simulink library "NeuroMuscularLibrary"  (R2014b)
settings: Solver=ode45  StartTime=0.0  StopTime=10.0  RelTol=1e-3
values from neighbouring files (symbols this model uses):
  c = 0.05    [BodyMechParams.m]
  c_jointstop = 0.3 / (pi/180)    (= 17.1887338539)    [BodyMechParams.m]
  DeltaThRef = 2e-3    (= 0.002)    [BodyMechParams.m]
  eref = 0.04    [BodyMechParams.m]
  footBallToAnkleDist = 0.16    [BodyMechParams.m]
  footBallToCenterDist = footLength/2    (= 0.1)    [BodyMechParams.m]
  footBallToHeelDist = footLength    (= 0.2)    [BodyMechParams.m]
  footCenterToCGDist = 0.14 - footBallToCenterDist    (= 0.04)    [BodyMechParams.m]
  footInertia = 0.005    [BodyMechParams.m]
  footLength = 0.2    [BodyMechParams.m]
  footMass = 1.25    [BodyMechParams.m]
  g = 9.80665    [BodyMechParams.m]
  groundTheta = [atan(diff(groundZ)./diff(groundX)), 0]    [generateGround.m]
  groundZ = groundZ * stepSize/(largestStep+eps)    [generateGround.m]
  hatHipToCenterDistLen = hatLength/2    (= 0.4)    [BodyMechParams.m]
  hatInertia = 3    [BodyMechParams.m]
  hatLeftHipToCenterDistWidth = .15    (= 0.15)    [BodyMechParams.m]
  hatLength = 0.8    [BodyMechParams.m]
  hatMass = 53.5    [BodyMechParams.m]
  hatThickness = 0.2    [BodyMechParams.m]
  hatWidth = 0.4    [BodyMechParams.m]
  K = 5    [BodyMechParams.m]
  k_gn = k_gz    (= 78453.2)    [BodyMechParams.m]
  k_gt = k_gz    (= 78453.2)    [BodyMechParams.m]
  k_pressure = hatMass * g / DeltaThRef    (= 262327.8875)    [BodyMechParams.m]
  loptGAS = 0.05    [BodyMechParams.m]
  loptGLU = 0.11    [BodyMechParams.m]
  loptHAM = 0.10    (= 0.1)    [BodyMechParams.m]
  loptHFL = 0.11    [BodyMechParams.m]
  loptSOL = 0.04    [BodyMechParams.m]
  loptTA = 0.06    [BodyMechParams.m]
  loptVAS = 0.08    [BodyMechParams.m]
  lslackGAS = 0.40    (= 0.4)    [BodyMechParams.m]
  lslackGLU = 0.13    [BodyMechParams.m]
  lslackHAM = 0.31    [BodyMechParams.m]
  lslackHFL = 0.10    (= 0.1)    [BodyMechParams.m]
  lslackSOL = 0.26    [BodyMechParams.m]
  lslackTA = 0.24    [BodyMechParams.m]
  lslackVAS = 0.23    [BodyMechParams.m]
  mu_slide = 0.8    [BodyMechParams.m]
  mu_stick = 0.9    [BodyMechParams.m]
  N = 1.5    [BodyMechParams.m]    (also in cmaes.m = size(x,1))
  phimaxGASa = 20*pi/180    (= 0.349065850399)    [BodyMechParams.m]
  phimaxGASk = 40*pi/180    (= 0.698131700798)    [BodyMechParams.m]
  phimaxHAMk = 0*pi/180    (= 0)    [BodyMechParams.m]
  phimaxSOL = 20*pi/180    (= 0.349065850399)    [BodyMechParams.m]
  phimaxTA = -10*pi/180    (= -0.174532925199)    [BodyMechParams.m]
  phimaxVAS = 15*pi/180    (= 0.261799387799)    [BodyMechParams.m]
  phirefGASa = -10*pi/180    (= -0.174532925199)    [BodyMechParams.m]
  phirefGASk = 15*pi/180    (= 0.261799387799)    [BodyMechParams.m]
  phirefGLU = -30*pi/180    (= -0.523598775598)    [BodyMechParams.m]
  phirefHAMh = -25*pi/180    (= -0.436332312999)    [BodyMechParams.m]
  phirefHAMk = 0*pi/180    (= 0)    [BodyMechParams.m]
  phirefHFL = 0*pi/180    (= 0)    [BodyMechParams.m]
  phirefSOL = -10*pi/180    (= -0.174532925199)    [BodyMechParams.m]
  phirefTA = 20*pi/180    (= 0.349065850399)    [BodyMechParams.m]
  phirefVAS = 55*pi/180    (= 0.959931088597)    [BodyMechParams.m]
  rGASa = 0.05    [BodyMechParams.m]
  rGASk = 0.05    [BodyMechParams.m]
  rGLU = 0.10    (= 0.1)    [BodyMechParams.m]
  rHAMh = 0.08    [BodyMechParams.m]
  rHAMk = 0.05    [BodyMechParams.m]
  rHFL = 0.10    (= 0.1)    [BodyMechParams.m]
  rhoGASa = 0.7    [BodyMechParams.m]
  rhoGASk = 0.7    [BodyMechParams.m]
  rhoGLU = 0.5    [BodyMechParams.m]
  rhoHAMh = 0.7    [BodyMechParams.m]
  rhoHAMk = 0.7    [BodyMechParams.m]
  rhoHFL = 0.5    [BodyMechParams.m]
  rhoSOL = 0.5    [BodyMechParams.m]
  rhoTA = 0.7    [BodyMechParams.m]
  rhoVAS = 0.7    [BodyMechParams.m]
  rSOL = 0.05    [BodyMechParams.m]
  rTA = 0.04    [BodyMechParams.m]
  rVAS = 0.06    [BodyMechParams.m]
  s = x(1:N-1,:).^2 + x(2:N,:).^2    [cmaes.m]
  shankAnkleToCenterDist = shankLength/2    (= 0.25)    [BodyMechParams.m]
  shankAnkleToKneeDist = shankLength    (= 0.5)    [BodyMechParams.m]
  shankCenterToCGDist = 0.3 - shankAnkleToCenterDist    (= 0.05)    [BodyMechParams.m]
  shankInertia = 0.05    [BodyMechParams.m]
  shankLength = 0.5    [BodyMechParams.m]
  shankMass = 3.5    [BodyMechParams.m]
  tau = 0.01    [BodyMechParams.m]
  thighCenterToCGDist = 0.3 - thighKneeToCenterDist    (= 0.05)    [BodyMechParams.m]
  thighInertia = 0.15    [BodyMechParams.m]
  thighKneeToCenterDist = thighLength/2    (= 0.25)    [BodyMechParams.m]
  thighKneeToHipDist = thighLength    (= 0.5)    [BodyMechParams.m]
  thighLength = 0.5    [BodyMechParams.m]
  thighMass = 8.5    [BodyMechParams.m]
  v_gn_max = v_gz_max    (= 0.03)    [BodyMechParams.m]
  v_gt_max = v_gz_max    (= 0.03)    [BodyMechParams.m]
  v_max_pressure = 0.5    [BodyMechParams.m]
  vLimit = 0.01    [BodyMechParams.m]
  w = 0.56    [BodyMechParams.m]    (also in cmaes.m = ones(size(x,1)))
  w_max_jointstop = 1 * pi/180    (= 0.0174532925199)    [BodyMechParams.m]
undefined symbols (not defined in the file or in its folder): ankleBackDriveGain, ankleDgain, ankleFilterPID, ankleFilterSEA, ankleGearEff, ankleGearRatio, ankleIgain, ankleInitialAngle, ankleInputMass, ankleParallelSpringDamping, ankleParallelSpringOffset, ankleParallelSpringStiffness, anklePgain, ankleSEADamping, ankleSEAStiffness, ankleTendonMass, deltaLegAngleThr, footMassp, FourBarL1, FourBarL3, GainGAS, GainGLU, GainHAM, GainKneeOverExt, GainSOL, GainSOLTA, GainTA, GainVAS, hipDGain, hipPGain, Kglu, kneeAngleOffset, kneeBackDriveGain, kneeDgain, kneeExtendGain, kneeFilterPID, kneeFilterSEA, kneeFlexGain, kneeGearEff, kneeGearRatio, kneeHoldGain1, kneeHoldGain2, kneeIgain, kneeInitialAngle, kneePgain, kneeSEADamping, kneeSEAStiffness, kneeStatorMass, kneeStopGain, legAngleFilter, legAngleSpeedMax, legLengthClr, motorBackEMF, motorInductance, motorMaxCurrent, motorMaxVoltage, motorResistance, motorRotorInertia, motorRotorMass, motorTorsionalConst ... (+19)
undefined symbols (not defined in the file): ankleCJointstop, ankleIntCoulomb, ankleIntDamping, ankleIntStatic, anklePlantarLimit, ankleWMaxJointstop, dryFrictionDamping, dryFrictionStiffness, dryFrictionVelThresh, FmaxGLU, FT_GLU, kneeCJointstop, kneeExtCoulomb, kneeExtDamping, kneeExtStatic, kneeIntCoulomb, kneeIntDamping, kneeIntStatic, kneeWMaxJointstop, phiKneeUpLimit, RGainGAS, RGainGLU, RGainHAM, RGainHAMCut, RGainKneeOverExt, RGainSOL, RGainSOLTA, RGainTA, RGainVAS, RhipDGain, RhipPGain, RKglu, RkneeExtendGain, RkneeFlexGain, RkneeHoldGain1, RkneeHoldGain2, RkneeStopGain, RlegAngleFilter, RlegLengthClr, RPosGainGG, RSpeedGainGG
libraries: sm_lib x90, nesl_utility x44, simulink x18, dspswit3 x10, NeuroMuscularLibrary x8, simulink_extras x2
(part 4 of 5)

== system NeuroMuscularLibrary/Full Prosthesis/Ankle SEA Control ==
  Motor Speed : Inport
  Load Acceleration : Inport  Port=2
  Measured Torque : Inport  Port=3
  Desired Ankle Torque : Inport  Port=4
  Parallel Spring Torque : Inport  Port=5
  Ankle Input Angle : Inport  Port=6
  Tendon Angle : Inport  Port=7
  Ankle Angle : Inport  Port=8
  4 bar ratio : Subsystem
  Divide : Product  Inputs=*/
  Feed Forward : Subsystem
  PID Controller : simulink/Continuous/PID Controller  Controller=PD  TimeDomain=Continuous-time  SampleTime=-1  IntegratorMethod=Forward Euler  FilterMethod=Forward Euler  Form=Parallel  P=anklePgain  I=ankleIgain  D=ankleDgain  N=ankleFilterPID  InitialConditionSource=internal  InitialConditionForIntegrator=0  InitialConditionForFilter=0  ExternalReset=none  LimitOutput=off  UpperSaturationLimit=inf  LowerSaturationLimit=-inf  LinearizeAsGain=on  AntiWindupMode=none  Kb=1  TrackingMode=off  Kt=1  PParamMin=[]  PParamMax=[]  IParamMin=[]  IParamMax=[]  DParamMin=[]  DParamMax=[]  NParamMin=[]  NParamMax=[]  KbParamMin=[]  KbParamMax=[]  KtParamMin=[]  KtParamMax=[]  POutMin=[]  POutMax=[]  IOutMin=[]  IOutMax=[]  DOutMin=[]  DOutMax=[]  NOutMin=[]  NOutMax=[]  KbOutMin=[]  KbOutMax=[]  KtOutMin=[]  KtOutMax=[]  IntegratorOutMin=[]  IntegratorOutMax=[]  FilterOutMin=[]  FilterOutMax=[]  SumOutMin=[]  SumOutMax=[]  SumI1OutMin=[]  SumI1OutMax=[]  SumI2OutMin=[]  SumI2OutMax=[]  SumI3OutMin=[]  SumI3OutMax=[]  SumDOutMin=[]  SumDOutMax=[]  SaturationOutMin=[]  SaturationOutMax=[]  IntegratorContinuousStateAttributes=''  IntegratorStateMustResolveToSignalObject=off  IntegratorRTWStateStorageClass=Auto  FilterContinuousStateAttributes=''  FilterStateMustResolveToSignalObject=off  FilterRTWStateStorageClass=Auto  DifferentiatorICPrevScaledInput=0  DifferentiatorOutMin=[]  DifferentiatorOutMax=[]  UseFilter=on
  Saturation1 : Saturate  UpperLimit=motorMaxVoltage  LowerLimit=-motorMaxVoltage  ZeroCross=off
  Sum : Sum  Inputs=|+-
  Sum1 : Sum  Inputs=+-|
  Sum2 : Sum  Inputs=|+-
  Motor Voltage : Outport
  Desired Actuator Torque : Outport  Port=2
  wires:
  Divide/1 -> Sum/1, Feed Forward/3(Desired Actuator Torque), Desired Actuator Torque/1  "Desired Actuator"
  Sum2/1 -> Divide/1
  Saturation1/1 -> Motor Voltage/1
  Sum1/1 -> Saturation1/1
  Load Acceleration/1 -> Feed Forward/2(Load Acceleration)
  Ankle Input Angle/1 -> 4 bar ratio/1(Ankle Input Angle)
  Tendon Angle/1 -> 4 bar ratio/2(Tendon Angle)
  Ankle Angle/1 -> 4 bar ratio/3(Ankle Angle)
  Measured Torque/1 -> Sum/2
  Sum/1 -> PID Controller/1
  4 bar ratio/1(ratio) -> Divide/2
  Motor Speed/1 -> Feed Forward/1(Motor Speed)
  Feed Forward/1(Computed Motor Voltage) -> Sum1/1
  Desired Ankle Torque/1 -> Sum2/1
  Parallel Spring Torque/1 -> Sum2/2
  PID Controller/1 -> Sum1/2

== system NeuroMuscularLibrary/Full Prosthesis/Ankle Tendon ==
  CG : sm_lib/Frames and Transforms/Reference Frame  BlockFunction=simmechanics.library.frames_transforms.reference_frame
  PS-Simulink Converter : nesl_utility/PS-Simulink Converter  PhysicalDomain=network_engine_domain  SubClassName=ps_output  LeftPortType=input  RightPortType=output  PseudoPeriodic=off  Frequencies=[]  Unit=1  AffineConversion=off
  Revolute Joint : sm_lib/Joints/Revolute Joint  SenseConstraintForce=off  SenseConstraintForceX=off  SenseConstraintForceY=off  SenseConstraintForceZ=off  SenseConstraintTorque=off  SenseConstraintTorqueX=off  SenseConstraintTorqueY=off  SenseConstraintTorqueZ=off  SenseTotalForce=off  SenseTotalForceX=off  SenseTotalForceY=off  SenseTotalForceZ=off  SenseTotalTorque=off  SenseTotalTorqueX=off  SenseTotalTorqueY=off  SenseTotalTorqueZ=off  CompositeWrenchDir=FollowerOnBase  CompositeWrenchFrame=BaseFrame  EquilibriumPosition=0  EquilibriumPositionUnits=deg  SpringStiffness=0  SpringStiffnessUnits=N*m/deg  DampingCoefficient=0  DampingCoefficientUnits=N*m/(deg/s)  TorqueActuationMode=NoTorque  MotionActuationMode=ComputedMotion  SensePosition=on  SenseVelocity=off  SenseAcceleration=off  SenseTorqueForce=off  PositionTargetValue=0  PositionTargetValueUnits=deg  PositionTargetSpecify=off  PositionTargetPriority=High  VelocityTargetValue=0  VelocityTargetValueUnits=deg/s  VelocityTargetSpecify=off  VelocityTargetPriority=High  BlockFunction=simmechanics.library.joints.revolute_joint
  Revolute Joint1 : sm_lib/Joints/Revolute Joint  SenseConstraintForce=off  SenseConstraintForceX=off  SenseConstraintForceY=off  SenseConstraintForceZ=off  SenseConstraintTorque=off  SenseConstraintTorqueX=off  SenseConstraintTorqueY=off  SenseConstraintTorqueZ=off  SenseTotalForce=off  SenseTotalForceX=off  SenseTotalForceY=off  SenseTotalForceZ=off  SenseTotalTorque=off  SenseTotalTorqueX=off  SenseTotalTorqueY=off  SenseTotalTorqueZ=off  CompositeWrenchDir=FollowerOnBase  CompositeWrenchFrame=BaseFrame  EquilibriumPosition=0  EquilibriumPositionUnits=deg  SpringStiffness=0  SpringStiffnessUnits=N*m/deg  DampingCoefficient=0  DampingCoefficientUnits=N*m/(deg/s)  TorqueActuationMode=NoTorque  MotionActuationMode=ComputedMotion  SensePosition=off  SenseVelocity=off  SenseAcceleration=off  SenseTorqueForce=off  PositionTargetValue=0  PositionTargetValueUnits=deg  PositionTargetSpecify=off  PositionTargetPriority=High  VelocityTargetValue=0  VelocityTargetValueUnits=deg/s  VelocityTargetSpecify=off  VelocityTargetPriority=High  BlockFunction=simmechanics.library.joints.revolute_joint
  Shank : sm_lib/Body Elements/Solid  InertiaType=Custom  Mass=ankleTendonMass  MassUnits=g  CenterOfMass=ankleTendonCG  CenterOfMassUnits=mm  MomentsOfInertia=ankleTendonMomentOfInertia  MomentsOfInertiaUnits=g*cm^2  ProductsOfInertia=ankleTendonProductOfInertia  ProductsOfInertiaUnits=g*cm^2  DensityBased=on  Density=1000  DensityUnits=kg/(m^3)  GraphicType=FromGeometry  MarkerShape=Sphere  MarkerSize=10  MarkerSizeUnits=m  GraphicVisPropType=SimpleVisualProperties  GraphicDiffuseColor=[0.5 0.5 0.5]  GraphicSpecularColor=[0.5 0.5 0.5 1.0]  GraphicAmbientColor=[0.15 0.15 0.15 1.0]  GraphicEmissiveColor=[0.0 0.0 0.0 1.0]  GraphicShininess=75  GraphicOpacity=1.0  GeometryShape=FromFile  RectangleSize=[1 1]  RectangleSizeUnits=m  BrickDimensions=[1 1 1]  BrickDimensionUnits=m  CylinderRadius=1  CylinderRadiusUnits=m  CylinderLength=1  CylinderLengthUnits=m  SphereRadius=1  SphereRadiusUnits=m  EllipsoidRadii=[1 1 1]  EllipsoidRadiiUnits=m  ExtrusionCrossSection=[1 1; -1 1; -1 -1; 1 -1]  ExtrusionCrossSectionUnits=m  ExtrusionLength=1  ExtrusionLengthUnits=m  PolygonNumSides=3  PolygonOuterRadius=1  PolygonOuterRadiusUnits=m  ExtGeomFileType=STL  ExtGeomFileName=ankleTendon.STL  ExtGeomFileUnits=mm  RevolutionCrossSection=[1 1; 1 -1; 2 -1; 2 1]  RevolutionCrossSectionUnits=m  RevolutionExtent=Full  RevolutionAngle=180  RevolutionAngleUnits=deg  BlockFunction=simmechanics.library.body_elements.solid
  To CG : sm_lib/Frames and Transforms/Rigid Transform  TranslationMethod=Cartesian  TranslationLengthUnit=mm  TranslationStandardAxis=-Z  TranslationStandardOffset=1.5  TranslationCartesianOffset=ankleTendonCG  TranslationROffset=0  TranslationROffsetUnits=m  TranslationZOffset=0  TranslationZOffsetUnits=m  TranslationThetaOffset=0  TranslationThetaOffsetUnits=deg  RotationMethod=None  RotationAngleUnits=deg  RotationStandardAxis=+Z  RotationAngle=0  RotationArbitraryAxis=[0 0 1]  FollAlignAxisA=+X  BaseAlignAxisA=+Y  FollAlignAxisB=+Y  BaseAlignAxisB=+Z  RotationMatrix=[1 0 0; 0 1 0; 0 0 1]  BlockFunction=simmechanics.library.frames_transforms.rigid_transform
  To Foot : sm_lib/Frames and Transforms/Rigid Transform  TranslationMethod=Cartesian  TranslationLengthUnit=mm  TranslationStandardAxis=-Y  TranslationStandardOffset=445.61  TranslationCartesianOffset=[0, -328.8, 0]  TranslationROffset=0  TranslationROffsetUnits=m  TranslationZOffset=0  TranslationZOffsetUnits=m  TranslationThetaOffset=0  TranslationThetaOffsetUnits=deg  RotationMethod=None  RotationAngleUnits=deg  RotationStandardAxis=+Z  RotationAngle=0  RotationArbitraryAxis=[0 0 1]  FollAlignAxisA=+X  BaseAlignAxisA=+Y  FollAlignAxisB=+Y  BaseAlignAxisB=+Z  RotationMatrix=[1 0 0; 0 1 0; 0 0 1]  BlockFunction=simmechanics.library.frames_transforms.rigid_transform
  " Ankle Input Joint" : PMIOPort  Port=1  Side=Left
  Foot : PMIOPort  Port=2  Side=Right
  Angle : Outport
  wires:
  PS-Simulink Converter/1 -> Angle/1
  connections:
  CG/RConn1 -- To CG/RConn1
  To Foot/LConn1 -- Revolute Joint/RConn1 -- To CG/LConn1 -- Shank/RConn1
  Revolute Joint/LConn1 -- " Ankle Input Joint"/RConn1
  Revolute Joint1/LConn1 -- To Foot/RConn1
  Foot/RConn1 -- Revolute Joint1/RConn1
  Revolute Joint/RConn2 -- PS-Simulink Converter/LConn1

== system NeuroMuscularLibrary/Full Prosthesis/Foot ==
  CG : sm_lib/Frames and Transforms/Reference Frame  BlockFunction=simmechanics.library.frames_transforms.reference_frame
  Shank : sm_lib/Body Elements/Solid  InertiaType=Custom  Mass=footMassp  MassUnits=g  CenterOfMass=footCG  CenterOfMassUnits=mm  MomentsOfInertia=footMomentOfInertia  MomentsOfInertiaUnits=g*cm^2  ProductsOfInertia=footProductOfInertia  ProductsOfInertiaUnits=g*cm^2  DensityBased=on  Density=1000  DensityUnits=kg/(m^3)  GraphicType=FromGeometry  MarkerShape=Sphere  MarkerSize=10  MarkerSizeUnits=m  GraphicVisPropType=SimpleVisualProperties  GraphicDiffuseColor=[0.5 0.5 0.5]  GraphicSpecularColor=[0.5 0.5 0.5 1.0]  GraphicAmbientColor=[0.15 0.15 0.15 1.0]  GraphicEmissiveColor=[0.0 0.0 0.0 1.0]  GraphicShininess=75  GraphicOpacity=1.0  GeometryShape=FromFile  RectangleSize=[1 1]  RectangleSizeUnits=m  BrickDimensions=[1 1 1]  BrickDimensionUnits=m  CylinderRadius=1  CylinderRadiusUnits=m  CylinderLength=1  CylinderLengthUnits=m  SphereRadius=1  SphereRadiusUnits=m  EllipsoidRadii=[1 1 1]  EllipsoidRadiiUnits=m  ExtrusionCrossSection=[1 1; -1 1; -1 -1; 1 -1]  ExtrusionCrossSectionUnits=m  ExtrusionLength=1  ExtrusionLengthUnits=m  PolygonNumSides=3  PolygonOuterRadius=1  PolygonOuterRadiusUnits=m  ExtGeomFileType=STL  ExtGeomFileName=foot.STL  ExtGeomFileUnits=mm  RevolutionCrossSection=[1 1; 1 -1; 2 -1; 2 1]  RevolutionCrossSectionUnits=m  RevolutionExtent=Full  RevolutionAngle=180  RevolutionAngleUnits=deg  BlockFunction=simmechanics.library.body_elements.solid
  To Ball : sm_lib/Frames and Transforms/Rigid Transform  TranslationMethod=Cartesian  TranslationLengthUnit=mm  TranslationStandardAxis=-Y  TranslationStandardOffset=445.61  TranslationCartesianOffset=[165, -63, 0]  TranslationROffset=0  TranslationROffsetUnits=m  TranslationZOffset=0  TranslationZOffsetUnits=m  TranslationThetaOffset=0  TranslationThetaOffsetUnits=deg  RotationMethod=None  RotationAngleUnits=deg  RotationStandardAxis=+Z  RotationAngle=0  RotationArbitraryAxis=[0 0 1]  FollAlignAxisA=+X  BaseAlignAxisA=+Y  FollAlignAxisB=+Y  BaseAlignAxisB=+Z  RotationMatrix=[1 0 0; 0 1 0; 0 0 1]  BlockFunction=simmechanics.library.frames_transforms.rigid_transform
  To CG : sm_lib/Frames and Transforms/Rigid Transform  TranslationMethod=Cartesian  TranslationLengthUnit=mm  TranslationStandardAxis=-Z  TranslationStandardOffset=1.5  TranslationCartesianOffset=footCG  TranslationROffset=0  TranslationROffsetUnits=m  TranslationZOffset=0  TranslationZOffsetUnits=m  TranslationThetaOffset=0  TranslationThetaOffsetUnits=deg  RotationMethod=None  RotationAngleUnits=deg  RotationStandardAxis=+Z  RotationAngle=0  RotationArbitraryAxis=[0 0 1]  FollAlignAxisA=+X  BaseAlignAxisA=+Y  FollAlignAxisB=+Y  BaseAlignAxisB=+Z  RotationMatrix=[1 0 0; 0 1 0; 0 0 1]  BlockFunction=simmechanics.library.frames_transforms.rigid_transform
  To Heel : sm_lib/Frames and Transforms/Rigid Transform  TranslationMethod=Cartesian  TranslationLengthUnit=mm  TranslationStandardAxis=-Y  TranslationStandardOffset=445.61  TranslationCartesianOffset=[-60, -63, 0]  TranslationROffset=0  TranslationROffsetUnits=m  TranslationZOffset=0  TranslationZOffsetUnits=m  TranslationThetaOffset=0  TranslationThetaOffsetUnits=deg  RotationMethod=None  RotationAngleUnits=deg  RotationStandardAxis=+Z  RotationAngle=0  RotationArbitraryAxis=[0 0 1]  FollAlignAxisA=+X  BaseAlignAxisA=+Y  FollAlignAxisB=+Y  BaseAlignAxisB=+Z  RotationMatrix=[1 0 0; 0 1 0; 0 0 1]  BlockFunction=simmechanics.library.frames_transforms.rigid_transform
  To Tendon : sm_lib/Frames and Transforms/Rigid Transform  TranslationMethod=Cartesian  TranslationLengthUnit=mm  TranslationStandardAxis=-Y  TranslationStandardOffset=445.61  TranslationCartesianOffset=[-81, -16.3, 0]  TranslationROffset=0  TranslationROffsetUnits=m  TranslationZOffset=0  TranslationZOffsetUnits=m  TranslationThetaOffset=0  TranslationThetaOffsetUnits=deg  RotationMethod=None  RotationAngleUnits=deg  RotationStandardAxis=+Z  RotationAngle=0  RotationArbitraryAxis=[0 0 1]  FollAlignAxisA=+X  BaseAlignAxisA=+Y  FollAlignAxisB=+Y  BaseAlignAxisB=+Z  RotationMatrix=[1 0 0; 0 1 0; 0 0 1]  BlockFunction=simmechanics.library.frames_transforms.rigid_transform
  " Ankle Input Joint" : PMIOPort  Port=1  Side=Right
  Tendon Bearing : PMIOPort  Port=2  Side=Left
  Ball : PMIOPort  Port=3  Side=Left
  Heel : PMIOPort  Port=4  Side=Right
  connections:
  Tendon Bearing/RConn1 -- To Tendon/RConn1
  CG/RConn1 -- To CG/RConn1
  To Tendon/LConn1 -- " Ankle Input Joint"/RConn1 -- Shank/RConn1 -- To CG/LConn1 -- To Heel/LConn1 -- To Ball/LConn1
  Ball/RConn1 -- To Ball/RConn1
  Heel/RConn1 -- To Heel/RConn1

== system NeuroMuscularLibrary/Full Prosthesis/Harmonic Drive// Series Elastic Actuator ==
  Motor Speed : Inport
  Motor Angle : Inport  Port=2
  Motor Torque : Inport  Port=3
  Load Angle : Inport  Port=4
  Load Speed : Inport  Port=5
  Add : Sum
  Damping : Gain  Gain=kneeSEADamping
  Gain : Gain  Gain=-1
  Mux : Mux  Inputs=2
  Ratio1 : Gain  Gain=1/kneeGearRatio
  Ratio2 : Gain  Gain=1/kneeGearRatio
  Ratio3 : Gain  Gain=1/kneeGearRatio
  Ratio4 : Gain  Gain=1/kneeGearEff
  Scope : Scope
  Stiffness : Gain  Gain=kneeSEAStiffness
  Sum : Sum  Inputs=|++
  Sum1 : Sum  Inputs=|++
  Sum2 : Sum  Inputs=++|
  Torque on Motor : Outport
  " Torque on Load" : Outport  Port=2
  wires:
  Mux/1 -> Scope/1
  Load Speed/1 -> Sum2/2
  Ratio3/1 -> Sum2/1
  Motor Torque/1 -> Sum1/2
  Ratio2/1 -> Ratio4/1
  Load Angle/1 -> Sum/1
  Add/1 -> Gain/1  "External Torque"
  Ratio1/1 -> Sum/2
  Sum1/1 -> Torque on Motor/1
  Stiffness/1 -> Add/2, Mux/1
  Sum/1 -> Stiffness/1
  Damping/1 -> Add/1, Mux/2
  Sum2/1 -> Damping/1
  Motor Speed/1 -> Ratio3/1
  Motor Angle/1 -> Ratio1/1
  Ratio4/1 -> Sum1/1
  Gain/1 -> " Torque on Load"/1, Ratio2/1

== system NeuroMuscularLibrary/Full Prosthesis/Harmonic Drive// Series Elastic Actuator1 ==
  Motor Speed : Inport
  Motor Angle : Inport  Port=2
  Motor Torque : Inport  Port=3
  Load Angle : Inport  Port=4
  Load Speed : Inport  Port=5
  Add : Sum
  Damping : Gain  Gain=ankleSEADamping
  Gain : Gain  Gain=-1
  Ratio1 : Gain  Gain=1/ankleGearRatio
  Ratio2 : Gain  Gain=1/ankleGearRatio
  Ratio3 : Gain  Gain=1/ankleGearRatio
  Ratio4 : Gain  Gain=1/ankleGearEff
  Stiffness : Gain  Gain=ankleSEAStiffness
  Sum : Sum  Inputs=|++
  Sum1 : Sum  Inputs=|++
  Sum2 : Sum  Inputs=++|
  Torque on Motor : Outport
  Torque on Load : Outport  Port=2
  wires:
  Gain/1 -> Torque on Load/1, Ratio2/1
  Load Speed/1 -> Sum2/2
  Ratio3/1 -> Sum2/1
  Motor Torque/1 -> Sum1/2
  Ratio2/1 -> Ratio4/1
  Load Angle/1 -> Sum/1
  Add/1 -> Gain/1  "External Torque"
  Ratio1/1 -> Sum/2
  Sum1/1 -> Torque on Motor/1
  Stiffness/1 -> Add/2
  Sum/1 -> Stiffness/1
  Damping/1 -> Add/1
  Sum2/1 -> Damping/1
  Motor Speed/1 -> Ratio3/1
  Motor Angle/1 -> Ratio1/1
  Ratio4/1 -> Sum1/1

== system NeuroMuscularLibrary/Full Prosthesis/Knee Joint ==
  External Torque : Inport
  Add : Sum  Inputs=+++
  Friction : Subsystem  Commented=on  mask{Fs=kneeExtStatic, Fc=kneeExtCoulomb, sigma0=dryFrictionStiffness, sigma1=dryFrictionDamping, v_s=dryFrictionVelThresh, Fv=kneeExtDamping}
      mask prompts: Fs "Static Friction"; Fc "Colulomb Friction"; sigma0 "Dry Friction Stiffness"; sigma1 "Dry Friction Damping"; v_s "Velocity Threshold"; Fv "Viscous Friction"
  Knee Joint : sm_lib/Joints/Revolute Joint  SenseConstraintForce=off  SenseConstraintForceX=off  SenseConstraintForceY=off  SenseConstraintForceZ=off  SenseConstraintTorque=off  SenseConstraintTorqueX=off  SenseConstraintTorqueY=off  SenseConstraintTorqueZ=off  SenseTotalForce=off  SenseTotalForceX=off  SenseTotalForceY=off  SenseTotalForceZ=off  SenseTotalTorque=off  SenseTotalTorqueX=off  SenseTotalTorqueY=off  SenseTotalTorqueZ=off  CompositeWrenchDir=FollowerOnBase  CompositeWrenchFrame=BaseFrame  EquilibriumPosition=0  EquilibriumPositionUnits=deg  SpringStiffness=0  SpringStiffnessUnits=N*m/rad  DampingCoefficient=0  DampingCoefficientUnits=N*m/(rad/s)  TorqueActuationMode=InputTorque  MotionActuationMode=ComputedMotion  SensePosition=on  SenseVelocity=on  SenseAcceleration=on  SenseTorqueForce=off  PositionTargetValue=kneeInitialAngle  PositionTargetValueUnits=rad  PositionTargetSpecify=on  PositionTargetPriority=High  VelocityTargetValue=0  VelocityTargetValueUnits=deg/s  VelocityTargetSpecify=off  VelocityTargetPriority=High  BlockFunction=simmechanics.library.joints.revolute_joint
  Knee Plantarflexion Limit : Subsystem  mask{phiUpLimit=0, ext=1, c_jointstop=kneeCJointstop, w_max_jointstop=kneeWMaxJointstop}
      mask prompts: phiUpLimit "Upper Limit [rad]"; ext "Extension values are positive or negative?"; c_jointstop "Stiffness"; w_max_jointstop "Max retraction speed"
      mask help:
      | This block implements a hard joint limit that will prevent the joint from extending past the specified upper limit.
      |
      | Used for the knee and hip joints.
  PS-Simulink Converter1 : nesl_utility/PS-Simulink Converter  PhysicalDomain=network_engine_domain  SubClassName=ps_output  LeftPortType=input  RightPortType=output  PseudoPeriodic=off  Frequencies=[]  Unit=rad/s^2  AffineConversion=off
  PS-Simulink Converter2 : nesl_utility/PS-Simulink Converter  PhysicalDomain=network_engine_domain  SubClassName=ps_output  LeftPortType=input  RightPortType=output  PseudoPeriodic=off  Frequencies=[]  Unit=rad  AffineConversion=off
  PS-Simulink Converter3 : nesl_utility/PS-Simulink Converter  PhysicalDomain=network_engine_domain  SubClassName=ps_output  LeftPortType=input  RightPortType=output  PseudoPeriodic=off  Frequencies=[]  Unit=rad/s  AffineConversion=off
  Scope : Scope  NumInputPorts=2
      settings: TimeRange=5  YMin=-0.5~-4  YMax=0.5~5  SaveName=ScopeData4
  Simulink-PS Converter : nesl_utility/Simulink-PS Converter  PhysicalDomain=network_engine_domain  SubClassName=ps_input  LeftPortType=input  RightPortType=output  PseudoPeriodic=off  Frequencies=[]  NoiseDistribution=none  NoiseParameters=[]  Unit=N*m  AffineConversion=off  InputFiltering=off  SimscapeFilterOrder=1  InputFilterTimeConstant=0.001  UdotUserProvided=1
  Knee Stator : PMIOPort  Port=1  Side=Right
  Shank : PMIOPort  Port=2  Side=Left
  Shank Angle : Outport
  Shank Speed : Outport  Port=2
  Shank Acceleration : Outport  Port=3
  Actual Torque : Outport  Port=4
  Knee Stop Torque : Outport  Port=5
  wires:
  Knee Plantarflexion Limit/1(M_stop [Nm]) -> Add/3, Knee Stop Torque/1
  PS-Simulink Converter2/1 -> Knee Plantarflexion Limit/1(phi [rad]), Shank Angle/1
  PS-Simulink Converter3/1 -> Knee Plantarflexion Limit/2(dphi [rad/s]), Scope/2, Friction/1(Velocity), Shank Speed/1
  PS-Simulink Converter1/1 -> Shank Acceleration/1
  Add/1 -> Actual Torque/1, Simulink-PS Converter/1
  External Torque/1 -> Add/1
  Friction/1(Friction Force) -> Add/2, Scope/1
  connections:
  Knee Joint/LConn1 -- Knee Stator/RConn1
  Knee Joint/RConn1 -- Shank/RConn1
  Knee Joint/RConn3 -- PS-Simulink Converter3/LConn1
  Knee Joint/RConn2 -- PS-Simulink Converter2/LConn1
  Knee Joint/LConn2 -- Simulink-PS Converter/RConn1
  Knee Joint/RConn4 -- PS-Simulink Converter1/LConn1

== system NeuroMuscularLibrary/Full Prosthesis/Knee Motor ==
  Voltage : Inport
  Net Motor Torque : Inport  Port=2
  Load Speed : Inport  Port=3
  Friction : Subsystem  Commented=on  mask{Fs=kneeIntStatic, Fc=kneeIntCoulomb, sigma0=dryFrictionStiffness, sigma1=dryFrictionDamping, v_s=dryFrictionVelThresh, Fv=kneeIntDamping}
      mask prompts: Fs "Static Friction"; Fc "Colulomb Friction"; sigma0 "Dry Friction Stiffness"; sigma1 "Dry Friction Damping"; v_s "Velocity Threshold"; Fv "Viscous Friction"
  Gain : Gain  Gain=-1
  Knee Motor Axis : sm_lib/Joints/Revolute Joint  SenseConstraintForce=off  SenseConstraintForceX=off  SenseConstraintForceY=off  SenseConstraintForceZ=off  SenseConstraintTorque=off  SenseConstraintTorqueX=off  SenseConstraintTorqueY=off  SenseConstraintTorqueZ=off  SenseTotalForce=off  SenseTotalForceX=off  SenseTotalForceY=off  SenseTotalForceZ=off  SenseTotalTorque=off  SenseTotalTorqueX=off  SenseTotalTorqueY=off  SenseTotalTorqueZ=off  CompositeWrenchDir=FollowerOnBase  CompositeWrenchFrame=BaseFrame  EquilibriumPosition=0  EquilibriumPositionUnits=deg  SpringStiffness=0  SpringStiffnessUnits=N*m/deg  DampingCoefficient=0  DampingCoefficientUnits=N*m/(deg/s)  TorqueActuationMode=InputTorque  MotionActuationMode=ComputedMotion  SensePosition=on  SenseVelocity=on  SenseAcceleration=off  SenseTorqueForce=off  PositionTargetValue=-kneeInitialAngle*kneeGearRatio  PositionTargetValueUnits=rad  PositionTargetSpecify=on  PositionTargetPriority=High  VelocityTargetValue=0  VelocityTargetValueUnits=deg/s  VelocityTargetSpecify=off  VelocityTargetPriority=High  BlockFunction=simmechanics.library.joints.revolute_joint
  Motor Dynamics : Subsystem
  PS-Simulink Converter : nesl_utility/PS-Simulink Converter  PhysicalDomain=network_engine_domain  SubClassName=ps_output  LeftPortType=input  RightPortType=output  PseudoPeriodic=off  Frequencies=[]  Unit=rad  AffineConversion=off
  PS-Simulink Converter1 : nesl_utility/PS-Simulink Converter  PhysicalDomain=network_engine_domain  SubClassName=ps_output  LeftPortType=input  RightPortType=output  PseudoPeriodic=off  Frequencies=[]  Unit=rad/s  AffineConversion=off
  Scope : Scope  NumInputPorts=2
      settings: TimeRange=5  YMin=-5~-0.2  YMax=4~0.2
  Simulink-PS Converter : nesl_utility/Simulink-PS Converter  PhysicalDomain=network_engine_domain  SubClassName=ps_input  LeftPortType=input  RightPortType=output  PseudoPeriodic=off  Frequencies=[]  NoiseDistribution=none  NoiseParameters=[]  Unit=N*m  AffineConversion=off  InputFiltering=off  SimscapeFilterOrder=1  InputFilterTimeConstant=0.001  UdotUserProvided=1
  Sum : Sum  Inputs=+|+
  Knee Stator : PMIOPort  Port=1  Side=Right
  Knee Rotor : PMIOPort  Port=2  Side=Left
  Motor Torque : Outport
  Motor Angle : Outport  Port=2
  Motor Speed : Outport  Port=3
  wires:
  Voltage/1 -> Motor Dynamics/1(Voltage)
  PS-Simulink Converter/1 -> Motor Angle/1
  PS-Simulink Converter1/1 -> Motor Dynamics/2(Speed), Motor Speed/1
  Sum/1 -> Motor Torque/1
  Motor Dynamics/1(Torque) -> Sum/1
  Friction/1(Friction Force) -> Sum/2, Scope/2
  Load Speed/1 -> Gain/1
  Gain/1 -> Friction/1(Velocity), Scope/1
  Net Motor Torque/1 -> Simulink-PS Converter/1
  connections:
  Knee Motor Axis/LConn1 -- Knee Stator/RConn1
  Knee Motor Axis/RConn2 -- PS-Simulink Converter/LConn1
  Knee Motor Axis/RConn3 -- PS-Simulink Converter1/LConn1
  Knee Motor Axis/LConn2 -- Simulink-PS Converter/RConn1
  Knee Motor Axis/RConn1 -- Knee Rotor/RConn1

== system NeuroMuscularLibrary/Full Prosthesis/Knee Motor Rotor ==
  CG : sm_lib/Frames and Transforms/Reference Frame  BlockFunction=simmechanics.library.frames_transforms.reference_frame
  Knee Rotor1 : sm_lib/Body Elements/Solid  InertiaType=Custom  Mass=motorRotorMass  MassUnits=g  CenterOfMass=motorRotorCG  CenterOfMassUnits=mm  MomentsOfInertia=motorRotorMomentOfInertia  MomentsOfInertiaUnits=g*cm^2  ProductsOfInertia=motorRotorProductOfInertia  ProductsOfInertiaUnits=g*cm^2  DensityBased=on  Density=1000  DensityUnits=kg/(m^3)  GraphicType=FromGeometry  MarkerShape=Sphere  MarkerSize=10  MarkerSizeUnits=m  GraphicVisPropType=SimpleVisualProperties  GraphicDiffuseColor=[0.5 0.5 0.5]  GraphicSpecularColor=[0.5 0.5 0.5 1.0]  GraphicAmbientColor=[0.15 0.15 0.15 1.0]  GraphicEmissiveColor=[0.0 0.0 0.0 1.0]  GraphicShininess=75  GraphicOpacity=1.0  GeometryShape=FromFile  RectangleSize=[1 1]  RectangleSizeUnits=m  BrickDimensions=[1 1 1]  BrickDimensionUnits=m  CylinderRadius=1  CylinderRadiusUnits=m  CylinderLength=1  CylinderLengthUnits=m  SphereRadius=1  SphereRadiusUnits=m  EllipsoidRadii=[1 1 1]  EllipsoidRadiiUnits=m  ExtrusionCrossSection=[1 1; -1 1; -1 -1; 1 -1]  ExtrusionCrossSectionUnits=m  ExtrusionLength=1  ExtrusionLengthUnits=m  PolygonNumSides=3  PolygonOuterRadius=1  PolygonOuterRadiusUnits=m  ExtGeomFileType=STL  ExtGeomFileName=motorRotor.STL  ExtGeomFileUnits=mm  RevolutionCrossSection=[1 1; 1 -1; 2 -1; 2 1]  RevolutionCrossSectionUnits=m  RevolutionExtent=Full  RevolutionAngle=180  RevolutionAngleUnits=deg  BlockFunction=simmechanics.library.body_elements.solid
  Rigid Transform : sm_lib/Frames and Transforms/Rigid Transform  TranslationMethod=StandardAxis  TranslationLengthUnit=mm  TranslationStandardAxis=+Z  TranslationStandardOffset=4.5  TranslationCartesianOffset=[0 0 0]  TranslationROffset=0  TranslationROffsetUnits=m  TranslationZOffset=0  TranslationZOffsetUnits=m  TranslationThetaOffset=0  TranslationThetaOffsetUnits=deg  RotationMethod=None  RotationAngleUnits=deg  RotationStandardAxis=+Z  RotationAngle=0  RotationArbitraryAxis=[0 0 1]  FollAlignAxisA=+X  BaseAlignAxisA=+Y  FollAlignAxisB=+Y  BaseAlignAxisB=+Z  RotationMatrix=[1 0 0; 0 1 0; 0 0 1]  BlockFunction=simmechanics.library.frames_transforms.rigid_transform
  ToCG : sm_lib/Frames and Transforms/Rigid Transform  TranslationMethod=Cartesian  TranslationLengthUnit=mm  TranslationStandardAxis=+Z  TranslationStandardOffset=0  TranslationCartesianOffset=motorRotorCG  TranslationROffset=0  TranslationROffsetUnits=m  TranslationZOffset=0  TranslationZOffsetUnits=m  TranslationThetaOffset=0  TranslationThetaOffsetUnits=deg  RotationMethod=None  RotationAngleUnits=deg  RotationStandardAxis=+Z  RotationAngle=0  RotationArbitraryAxis=[0 0 1]  FollAlignAxisA=+X  BaseAlignAxisA=+Y  FollAlignAxisB=+Y  BaseAlignAxisB=+Z  RotationMatrix=[1 0 0; 0 1 0; 0 0 1]  BlockFunction=simmechanics.library.frames_transforms.rigid_transform
  Conn1 : PMIOPort  Port=1  Side=Right
  connections:
  CG/RConn1 -- ToCG/RConn1
  ToCG/LConn1 -- Knee Rotor1/RConn1 -- Rigid Transform/RConn1
  Conn1/RConn1 -- Rigid Transform/LConn1

== system NeuroMuscularLibrary/Full Prosthesis/Knee SEA Control ==
  Motor Speed : Inport
  Load Acceleration : Inport  Port=2
  Measured Torque : Inport  Port=3
  Desired Torque : Inport  Port=4
  Feed Forward : Subsystem
  PID Controller : simulink/Continuous/PID Controller  Controller=PD  TimeDomain=Continuous-time  SampleTime=-1  IntegratorMethod=Forward Euler  FilterMethod=Forward Euler  Form=Parallel  P=kneePgain  I=kneeIgain  D=kneeDgain  N=kneeFilterPID  InitialConditionSource=internal  InitialConditionForIntegrator=0  InitialConditionForFilter=0  ExternalReset=none  LimitOutput=off  UpperSaturationLimit=inf  LowerSaturationLimit=-inf  LinearizeAsGain=on  AntiWindupMode=none  Kb=1  TrackingMode=off  Kt=1  PParamMin=[]  PParamMax=[]  IParamMin=[]  IParamMax=[]  DParamMin=[]  DParamMax=[]  NParamMin=[]  NParamMax=[]  KbParamMin=[]  KbParamMax=[]  KtParamMin=[]  KtParamMax=[]  POutMin=[]  POutMax=[]  IOutMin=[]  IOutMax=[]  DOutMin=[]  DOutMax=[]  NOutMin=[]  NOutMax=[]  KbOutMin=[]  KbOutMax=[]  KtOutMin=[]  KtOutMax=[]  IntegratorOutMin=[]  IntegratorOutMax=[]  FilterOutMin=[]  FilterOutMax=[]  SumOutMin=[]  SumOutMax=[]  SumI1OutMin=[]  SumI1OutMax=[]  SumI2OutMin=[]  SumI2OutMax=[]  SumI3OutMin=[]  SumI3OutMax=[]  SumDOutMin=[]  SumDOutMax=[]  SaturationOutMin=[]  SaturationOutMax=[]  IntegratorContinuousStateAttributes=''  IntegratorStateMustResolveToSignalObject=off  IntegratorRTWStateStorageClass=Auto  FilterContinuousStateAttributes=''  FilterStateMustResolveToSignalObject=off  FilterRTWStateStorageClass=Auto  DifferentiatorICPrevScaledInput=0  DifferentiatorOutMin=[]  DifferentiatorOutMax=[]  UseFilter=on
  Saturation1 : Saturate  UpperLimit=motorMaxVoltage  LowerLimit=-motorMaxVoltage  ZeroCross=off
  Sum : Sum  Inputs=|+-
  Sum1 : Sum  Inputs=+-|
  Motor Voltage : Outport
  wires:
  Saturation1/1 -> Motor Voltage/1
  Sum1/1 -> Saturation1/1
  Load Acceleration/1 -> Feed Forward/2(Load Acceleration)
  Measured Torque/1 -> Sum/2  "Meaasured Torque"
  Desired Torque/1 -> Feed Forward/3(Desired Torque), Sum/1
  Sum/1 -> PID Controller/1
  Motor Speed/1 -> Feed Forward/1(Motor Speed)
  Feed Forward/1(Computed Motor Voltage) -> Sum1/1
  PID Controller/1 -> Sum1/2

== system NeuroMuscularLibrary/Full Prosthesis/Knee Stator ==
  CG : sm_lib/Frames and Transforms/Reference Frame  BlockFunction=simmechanics.library.frames_transforms.reference_frame
  Knee Stator Solid : sm_lib/Body Elements/Solid  InertiaType=Custom  Mass=kneeStatorMass  MassUnits=g  CenterOfMass=kneeStatorCG  CenterOfMassUnits=mm  MomentsOfInertia=kneeStatorMomentOfInertia  MomentsOfInertiaUnits=g*cm^2  ProductsOfInertia=kneeStatorProductOfInertia  ProductsOfInertiaUnits=g*cm^2  DensityBased=off  Density=1000  DensityUnits=kg/(m^3)  GraphicType=FromGeometry  MarkerShape=Sphere  MarkerSize=10  MarkerSizeUnits=m  GraphicVisPropType=SimpleVisualProperties  GraphicDiffuseColor=[0.5 0.5 0.5]  GraphicSpecularColor=[0.5 0.5 0.5 1.0]  GraphicAmbientColor=[0.15 0.15 0.15 1.0]  GraphicEmissiveColor=[0.0 0.0 0.0 1.0]  GraphicShininess=75  GraphicOpacity=1  GeometryShape=FromFile  RectangleSize=[1 1]  RectangleSizeUnits=m  BrickDimensions=[1 1 1]  BrickDimensionUnits=m  CylinderRadius=1  CylinderRadiusUnits=m  CylinderLength=1  CylinderLengthUnits=m  SphereRadius=1  SphereRadiusUnits=m  EllipsoidRadii=[1 1 1]  EllipsoidRadiiUnits=m  ExtrusionCrossSection=[1 1; -1 1; -1 -1; 1 -1]  ExtrusionCrossSectionUnits=m  ExtrusionLength=1  ExtrusionLengthUnits=m  PolygonNumSides=3  PolygonOuterRadius=1  PolygonOuterRadiusUnits=m  ExtGeomFileType=STL  ExtGeomFileName=kneeStator.STL  ExtGeomFileUnits=mm  RevolutionCrossSection=[1 1; 1 -1; 2 -1; 2 1]  RevolutionCrossSectionUnits=m  RevolutionExtent=Full  RevolutionAngle=180  RevolutionAngleUnits=deg  BlockFunction=simmechanics.library.body_elements.solid
  Rigid Transform : sm_lib/Frames and Transforms/Rigid Transform  TranslationMethod=Cartesian  TranslationLengthUnit=mm  TranslationStandardAxis=+Z  TranslationStandardOffset=0  TranslationCartesianOffset=[0, 0, -2]  TranslationROffset=0  TranslationROffsetUnits=m  TranslationZOffset=0  TranslationZOffsetUnits=m  TranslationThetaOffset=0  TranslationThetaOffsetUnits=deg  RotationMethod=None  RotationAngleUnits=deg  RotationStandardAxis=+Z  RotationAngle=0  RotationArbitraryAxis=[0 0 1]  FollAlignAxisA=+X  BaseAlignAxisA=+Y  FollAlignAxisB=+Y  BaseAlignAxisB=+Z  RotationMatrix=[1 0 0; 0 1 0; 0 0 1]  BlockFunction=simmechanics.library.frames_transforms.rigid_transform
  To CG : sm_lib/Frames and Transforms/Rigid Transform  TranslationMethod=Cartesian  TranslationLengthUnit=mm  TranslationStandardAxis=+Z  TranslationStandardOffset=0  TranslationCartesianOffset=kneeStatorCG  TranslationROffset=0  TranslationROffsetUnits=m  TranslationZOffset=0  TranslationZOffsetUnits=m  TranslationThetaOffset=0  TranslationThetaOffsetUnits=deg  RotationMethod=None  RotationAngleUnits=deg  RotationStandardAxis=+Z  RotationAngle=0  RotationArbitraryAxis=[0 0 1]  FollAlignAxisA=+Y  BaseAlignAxisA=+Z  FollAlignAxisB=+X  BaseAlignAxisB=+X  RotationMatrix=[1 0 0; 0 1 0; 0 0 1]  BlockFunction=simmechanics.library.frames_transforms.rigid_transform
  Thigh : PMIOPort  Port=1  Side=Right
  Knee Stator : PMIOPort  Port=2  Side=Left
  connections:
  CG/RConn1 -- To CG/RConn1
  To CG/LConn1 -- Knee Stator Solid/RConn1 -- Knee Stator/RConn1 -- Rigid Transform/RConn1
  Rigid Transform/LConn1 -- Thigh/RConn1

== system NeuroMuscularLibrary/Full Prosthesis/Shank ==
  CG : sm_lib/Frames and Transforms/Reference Frame  BlockFunction=simmechanics.library.frames_transforms.reference_frame
  Shank : sm_lib/Body Elements/Solid  InertiaType=Custom  Mass=shankMassp  MassUnits=g  CenterOfMass=shankCG  CenterOfMassUnits=mm  MomentsOfInertia=shankMomentOfInertia  MomentsOfInertiaUnits=g*cm^2  ProductsOfInertia=shankProductOfInertia  ProductsOfInertiaUnits=g*cm^2  DensityBased=on  Density=1000  DensityUnits=kg/(m^3)  GraphicType=FromGeometry  MarkerShape=Sphere  MarkerSize=10  MarkerSizeUnits=m  GraphicVisPropType=SimpleVisualProperties  GraphicDiffuseColor=[0.5 0.5 0.5]  GraphicSpecularColor=[0.5 0.5 0.5 1.0]  GraphicAmbientColor=[0.15 0.15 0.15 1.0]  GraphicEmissiveColor=[0.0 0.0 0.0 1.0]  GraphicShininess=75  GraphicOpacity=1.0  GeometryShape=FromFile  RectangleSize=[1 1]  RectangleSizeUnits=m  BrickDimensions=[1 1 1]  BrickDimensionUnits=m  CylinderRadius=1  CylinderRadiusUnits=m  CylinderLength=1  CylinderLengthUnits=m  SphereRadius=1  SphereRadiusUnits=m  EllipsoidRadii=[1 1 1]  EllipsoidRadiiUnits=m  ExtrusionCrossSection=[1 1; -1 1; -1 -1; 1 -1]  ExtrusionCrossSectionUnits=m  ExtrusionLength=1  ExtrusionLengthUnits=m  PolygonNumSides=3  PolygonOuterRadius=1  PolygonOuterRadiusUnits=m  ExtGeomFileType=STL  ExtGeomFileName=shankwKneeSEA.STL  ExtGeomFileUnits=mm  RevolutionCrossSection=[1 1; 1 -1; 2 -1; 2 1]  RevolutionCrossSectionUnits=m  RevolutionExtent=Full  RevolutionAngle=180  RevolutionAngleUnits=deg  BlockFunction=simmechanics.library.body_elements.solid
  To Ankle Stator : sm_lib/Frames and Transforms/Rigid Transform  TranslationMethod=StandardAxis  TranslationLengthUnit=mm  TranslationStandardAxis=-Y  TranslationStandardOffset=124.50  TranslationCartesianOffset=[0 0 0]  TranslationROffset=0  TranslationROffsetUnits=m  TranslationZOffset=0  TranslationZOffsetUnits=m  TranslationThetaOffset=0  TranslationThetaOffsetUnits=deg  RotationMethod=None  RotationAngleUnits=deg  RotationStandardAxis=+Z  RotationAngle=0  RotationArbitraryAxis=[0 0 1]  FollAlignAxisA=+Z  BaseAlignAxisA=+Y  FollAlignAxisB=+Y  BaseAlignAxisB=+Z  RotationMatrix=[1 0 0; 0 1 0; 0 0 1]  BlockFunction=simmechanics.library.frames_transforms.rigid_transform
  To CG : sm_lib/Frames and Transforms/Rigid Transform  TranslationMethod=Cartesian  TranslationLengthUnit=mm  TranslationStandardAxis=-Z  TranslationStandardOffset=1.5  TranslationCartesianOffset=shankCG  TranslationROffset=0  TranslationROffsetUnits=m  TranslationZOffset=0  TranslationZOffsetUnits=m  TranslationThetaOffset=0  TranslationThetaOffsetUnits=deg  RotationMethod=None  RotationAngleUnits=deg  RotationStandardAxis=+Z  RotationAngle=0  RotationArbitraryAxis=[0 0 1]  FollAlignAxisA=+X  BaseAlignAxisA=+Y  FollAlignAxisB=+Y  BaseAlignAxisB=+Z  RotationMatrix=[1 0 0; 0 1 0; 0 0 1]  BlockFunction=simmechanics.library.frames_transforms.rigid_transform
  To Foot : sm_lib/Frames and Transforms/Rigid Transform  TranslationMethod=Cartesian  TranslationLengthUnit=mm  TranslationStandardAxis=-Y  TranslationStandardOffset=445.61  TranslationCartesianOffset=[0, -436.9988, 2]  TranslationROffset=0  TranslationROffsetUnits=m  TranslationZOffset=0  TranslationZOffsetUnits=m  TranslationThetaOffset=0  TranslationThetaOffsetUnits=deg  RotationMethod=None  RotationAngleUnits=deg  RotationStandardAxis=+Z  RotationAngle=0  RotationArbitraryAxis=[0 0 1]  FollAlignAxisA=+X  BaseAlignAxisA=+Y  FollAlignAxisB=+Y  BaseAlignAxisB=+Z  RotationMatrix=[1 0 0; 0 1 0; 0 0 1]  BlockFunction=simmechanics.library.frames_transforms.rigid_transform
  Knee Stator : PMIOPort  Port=1  Side=Right
  Ankle Stator : PMIOPort  Port=2  Side=Left
  Ankle : PMIOPort  Port=3  Side=Left
  connections:
  Ankle/RConn1 -- To Foot/RConn1
  CG/RConn1 -- To CG/RConn1
  Ankle Stator/RConn1 -- To Ankle Stator/RConn1
  To Foot/LConn1 -- Knee Stator/RConn1 -- To Ankle Stator/LConn1 -- To CG/LConn1 -- Shank/RConn1

== system NeuroMuscularLibrary/Ground Contact Model/2D Contact ==
  RefPt [m m] : Inport
  nVec [m m] : Inport  Port=2
  pVec [m m] : Inport  Port=3
  vVec [m/s m/s] : Inport  Port=4
  Contact! : EnablePort  StatesWhenEnabling=reset
  Friction Switch : Subsystem
  Kinetic Friction Model : Subsystem
  Logical Operator : Logic  Operator=NOT  AllPortsSameDT=off  OutDataTypeStr=boolean
  Static Friction Model : Subsystem
  Sum : Sum
  Sum1 : Sum
  FnVec [N N] : Outport  OutputWhenDisabled=reset  InitialOutput=[0 0]
      settings: AttributesFormatString=when disabled: %<OutputWhenDisabled>
  FtVec [N N] : Outport  Port=2  OutputWhenDisabled=reset  InitialOutput=[0 0]
      settings: AttributesFormatString=when disabled: %<OutputWhenDisabled>
  wires:
  Kinetic Friction Model/1(RefPtFP [m m]) -> Static Friction Model/3(RefPtFP [m m])
  Kinetic Friction Model/3(nVec FP [m m]) -> Static Friction Model/5(nVecFP [m m])
  RefPt [m m]/1 -> Kinetic Friction Model/3(RefPt [m m])
  Static Friction Model/3(Sliding!) -> Friction Switch/1(Slide!)
  Sum/1 -> FtVec [N N]/1  "F_tVec"
  Sum1/1 -> FnVec [N N]/1  "F_nVec"
  Static Friction Model/2(F_t Stick [N N]) -> Sum/1
  Kinetic Friction Model/5(F_t Slide [N N]) -> Sum/2
  Kinetic Friction Model/6(F_n Slide [N N]) -> Sum1/2
  Static Friction Model/1(F_n Stick [N N]) -> Sum1/1
  Kinetic Friction Model/4(Stiction!) -> Friction Switch/2(Stick!)
  nVec [m m]/1 -> Kinetic Friction Model/4(nVec [m m])
  Friction Switch/1(Stiction) -> Logical Operator/1, Static Friction Model/Enable
  Kinetic Friction Model/2(posFP [m m]) -> Static Friction Model/4(posFP [m])
  vVec [m/s m/s]/1 -> Kinetic Friction Model/1(vel [m/s m/s]), Static Friction Model/2(vel [m/s m/s])
  pVec [m m]/1 -> Kinetic Friction Model/2(pos [m m]), Static Friction Model/1(pos [m])
  Logical Operator/1 -> Kinetic Friction Model/Enable

== system NeuroMuscularLibrary/Ground Height Lookup/Env Lookup ==
  x : Inport
  Gain : Gain  Gain=-1
  Ground Slope : Interpolation_n-D  NumberOfTableDimensions=1  Table=groundTheta  InterpMethod=Flat
      settings: InputPortMap=u0,u1
  Ground Z : Interpolation_n-D  NumberOfTableDimensions=1  Table=groundZ
      settings: InputPortMap=u0,u1
  Mux8 : Mux  Inputs=5
  Prelookup : PreLookup  BreakpointsData=groundX  BeginIndexSearchUsingPreviousIndexResult=on  ExtrapMethod=Linear  RndMeth=Simplest
  Trigonometric Function1 : Trigonometry
  Trigonometric Function2 : Trigonometry  Operator=cos
  Env : Outport
  wires:
  Prelookup/2 -> Ground Slope/2, Ground Z/2
  Trigonometric Function1/1 -> Gain/1
  Gain/1 -> Mux8/4
  Ground Slope/1 -> Trigonometric Function1/1, Trigonometric Function2/1
  Prelookup/1 -> Ground Slope/1, Ground Z/1
  Trigonometric Function2/1 -> Mux8/5
  x/1 -> Mux8/2, Prelookup/1
  Ground Z/1 -> Mux8/3, Mux8/1
  Mux8/1 -> Env/1

== system NeuroMuscularLibrary/Ground Height Lookup/Env Lookup1 ==
  x : Inport
  Gain : Gain  Gain=-1
  Ground Slope : Interpolation_n-D  NumberOfTableDimensions=1  Table=groundTheta  InterpMethod=Flat
      settings: InputPortMap=u0,u1
  Ground Z : Interpolation_n-D  NumberOfTableDimensions=1  Table=groundZ
      settings: InputPortMap=u0,u1
  Mux8 : Mux  Inputs=5
  Prelookup : PreLookup  BreakpointsData=groundX  BeginIndexSearchUsingPreviousIndexResult=on  ExtrapMethod=Linear  RndMeth=Simplest
  Trigonometric Function1 : Trigonometry
  Trigonometric Function2 : Trigonometry  Operator=cos
  Env : Outport
  wires:
  Prelookup/2 -> Ground Slope/2, Ground Z/2
  Trigonometric Function1/1 -> Gain/1
  Gain/1 -> Mux8/4
  Ground Slope/1 -> Trigonometric Function1/1, Trigonometric Function2/1
  Prelookup/1 -> Ground Slope/1, Ground Z/1
  Trigonometric Function2/1 -> Mux8/5
  x/1 -> Mux8/2, Prelookup/1
  Ground Z/1 -> Mux8/3, Mux8/1
  Mux8/1 -> Env/1

== system NeuroMuscularLibrary/Ground Height Lookup/Env Lookup2 ==
  x : Inport
  Gain : Gain  Gain=-1
  Ground Slope : Interpolation_n-D  NumberOfTableDimensions=1  Table=groundTheta  InterpMethod=Flat
      settings: InputPortMap=u0,u1
  Ground Z : Interpolation_n-D  NumberOfTableDimensions=1  Table=groundZ
      settings: InputPortMap=u0,u1
  Mux8 : Mux  Inputs=5
  Prelookup : PreLookup  BreakpointsData=groundX  BeginIndexSearchUsingPreviousIndexResult=on  ExtrapMethod=Linear  RndMeth=Simplest
  Trigonometric Function1 : Trigonometry
  Trigonometric Function2 : Trigonometry  Operator=cos
  Env : Outport
  wires:
  Prelookup/2 -> Ground Slope/2, Ground Z/2
  Trigonometric Function1/1 -> Gain/1
  Gain/1 -> Mux8/4
  Ground Slope/1 -> Trigonometric Function1/1, Trigonometric Function2/1
  Prelookup/1 -> Ground Slope/1, Ground Z/1
  Trigonometric Function2/1 -> Mux8/5
  x/1 -> Mux8/2, Prelookup/1
  Ground Z/1 -> Mux8/3, Mux8/1
  Mux8/1 -> Env/1

== system NeuroMuscularLibrary/Ground Height Lookup/Env Lookup3 ==
  x : Inport
  Gain : Gain  Gain=-1
  Ground Slope : Interpolation_n-D  NumberOfTableDimensions=1  Table=groundTheta  InterpMethod=Flat
      settings: InputPortMap=u0,u1
  Ground Z : Interpolation_n-D  NumberOfTableDimensions=1  Table=groundZ
      settings: InputPortMap=u0,u1
  Mux8 : Mux  Inputs=5
  Prelookup : PreLookup  BreakpointsData=groundX  BeginIndexSearchUsingPreviousIndexResult=on  ExtrapMethod=Linear  RndMeth=Simplest
  Trigonometric Function1 : Trigonometry
  Trigonometric Function2 : Trigonometry  Operator=cos
  Env : Outport
  wires:
  Prelookup/2 -> Ground Slope/2, Ground Z/2
  Trigonometric Function1/1 -> Gain/1
  Gain/1 -> Mux8/4
  Ground Slope/1 -> Trigonometric Function1/1, Trigonometric Function2/1
  Prelookup/1 -> Ground Slope/1, Ground Z/1
  Trigonometric Function2/1 -> Mux8/5
  x/1 -> Mux8/2, Prelookup/1
  Ground Z/1 -> Mux8/3, Mux8/1
  Mux8/1 -> Env/1

== system NeuroMuscularLibrary/Ground Height Lookup/Env Lookup4 ==
  x : Inport
  Gain : Gain  Gain=-1
  Ground Slope : Interpolation_n-D  NumberOfTableDimensions=1  Table=groundTheta  InterpMethod=Flat
      settings: InputPortMap=u0,u1
  Ground Z : Interpolation_n-D  NumberOfTableDimensions=1  Table=groundZ
      settings: InputPortMap=u0,u1
  Mux8 : Mux  Inputs=5
  Prelookup : PreLookup  BreakpointsData=groundX  BeginIndexSearchUsingPreviousIndexResult=on  ExtrapMethod=Linear  RndMeth=Simplest
  Trigonometric Function1 : Trigonometry
  Trigonometric Function2 : Trigonometry  Operator=cos
  Env : Outport
  wires:
  Prelookup/2 -> Ground Slope/2, Ground Z/2
  Trigonometric Function1/1 -> Gain/1
  Gain/1 -> Mux8/4
  Ground Slope/1 -> Trigonometric Function1/1, Trigonometric Function2/1
  Prelookup/1 -> Ground Slope/1, Ground Z/1
  Trigonometric Function2/1 -> Mux8/5
  x/1 -> Mux8/2, Prelookup/1
  Ground Z/1 -> Mux8/3, Mux8/1
  Mux8/1 -> Env/1
